simulink model "Pr_1"  (R2024a)
settings: Solver=VariableStepAuto  StartTime=0.0  StopTime=50  RelTol=1e-3
settings Model: Creator=user  LastModifiedBy=user

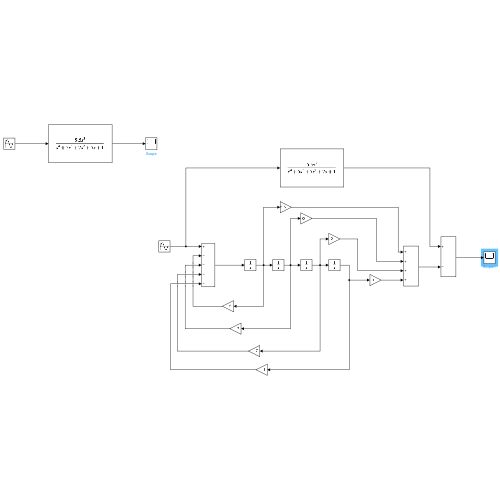
[thumbnail: Simulink's stored preview of the top-level diagram]
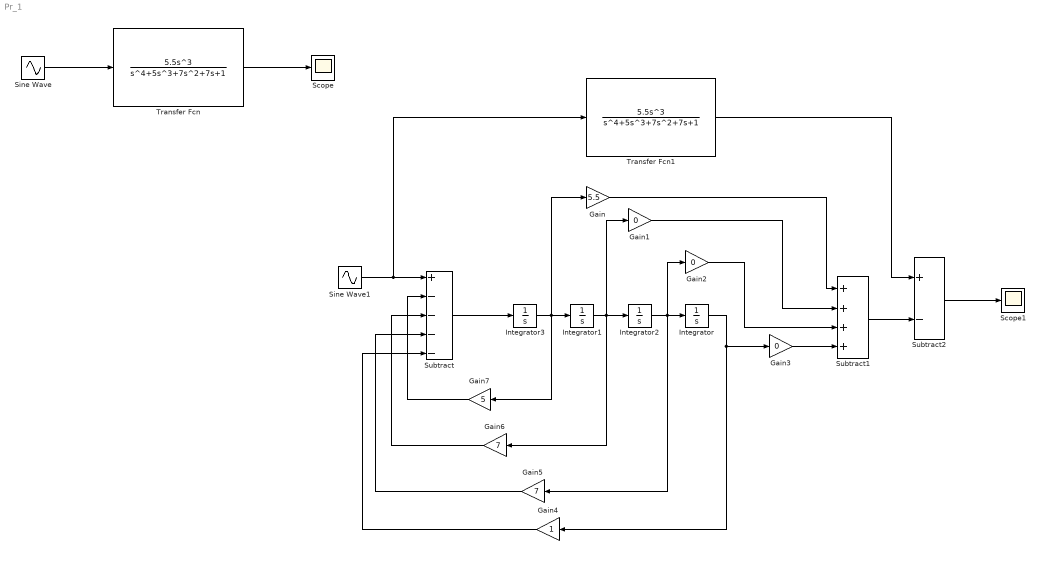
== system Pr_1 ==
  Gain : Gain  Gain=5.5
  Gain1 : Gain  Gain=0
  Gain2 : Gain  Gain=0
  Gain3 : Gain  Gain=0
  Gain4 : Gain
  Gain5 : Gain  Gain=7
  Gain6 : Gain  Gain=7
  Gain7 : Gain  Gain=5
  Integrator{,1..3} (4 alike) : Integrator
  Scope : Scope
  Scope1 : Scope
  Sine Wave : Sin  SampleTime=0
  Sine Wave1 : Sin  SampleTime=0
  Subtract : Sum  Inputs=+----
  Subtract1 : Sum  Inputs=++++
  Subtract2 : Sum  Inputs=+-
  Transfer Fcn : TransferFcn  Numerator=[5.5 0 0 0]  Denominator=[1 5 7 7 1]
  Transfer Fcn1 : TransferFcn  Numerator=[5.5 0 0 0]  Denominator=[1 5 7 7 1]
  wires:
  Sine Wave/1 -> Transfer Fcn/1
  Transfer Fcn/1 -> Scope/1
  Sine Wave1/1 -> Transfer Fcn1/1, Subtract/1
  Integrator2/1 -> Gain2/1, Gain5/1, Integrator/1
  Integrator3/1 -> Gain/1, Gain7/1, Integrator1/1
  Integrator1/1 -> Gain1/1, Gain6/1, Integrator2/1
  Subtract/1 -> Integrator3/1
  Gain7/1 -> Subtract/2
  Gain6/1 -> Subtract/3
  Gain5/1 -> Subtract/4
  Gain4/1 -> Subtract/5
  Integrator/1 -> Gain3/1, Gain4/1
  Gain/1 -> Subtract1/1
  Gain1/1 -> Subtract1/2
  Gain2/1 -> Subtract1/3
  Gain3/1 -> Subtract1/4
  Subtract1/1 -> Subtract2/2
  Transfer Fcn1/1 -> Subtract2/1
  Subtract2/1 -> Scope1/1
